simulink model "mCounterWithSaturation"  (R2021b)
settings: Solver=FixedStepAuto  StartTime=0.0  StopTime=10.0  RelTol=1e-3
PreLoadFcn:
  | A=1;B=1;C=2;D=1;
CloseFcn:
  | clear A B C D;
settings Model: Creator=nrangava  LastModifiedBy=nrangava
settings SolverCC: AlgebraicLoopSolver=TrustRegion  MaxZcPerStep=1
settings DataIOCC: SaveFormat=StructureWithTime  SaveState=on  DSMLogging=off  OutputSaveName=yout1,yout2
settings OptimizationCC: DefaultParameterBehavior=Inlined  EnhancedBackFolding=on  PassReuseOutputArgsAs=Individual arguments  ZeroExternalMemoryAtStartup=off  ZeroInternalMemoryAtStartup=off  OptimizeBlockOrder=speed  DifferentSizesBufferReuse=on  OptimizationCustomize=off  EfficientTunableParamExpr=on
settings DebuggingCC: ParameterTunabilityLossMsg=error  SFMachineParentedDataDiag=warning
settings HardwareCC: TargetBitPerPointer=64  TargetBitPerSizeT=64  TargetBitPerPtrDiffT=64  TargetLongLongMode=on  TargetIntDivRoundTo=Zero  TargetEndianess=LittleEndian  TargetWordSize=64  TargetHWDeviceType=Custom Processor->MATLAB Host Computer  ProdEqTarget=off
settings ModelReferenceCC: UpdateModelReferenceTargets=IfOutOfDate
settings SFSimCC: MATLABDynamicMemAlloc=off
settings RTWCC: Description=Embedded Coder  SystemTargetFile=ert.tlc  TemplateMakefile=ert_default_tmf  RTWVerbose=off  RetainRTWFile=on  TLCAssert=on
settings CodeAppCC: ForceParamTrailComments=on  IgnoreCustomStorageClasses=off  MaxIdLength=64  OperatorAnnotations=on  SimulinkDataObjDesc=on  SFDataObjDesc=on  InsertBlockDesc=on
settings ERTTargetCC: TargetLangStandard=C99 (ISO)  GenerateSampleERTMain=on  CombineOutputUpdateFcns=off  LogVarNameModifier=none  MatFileLogging=on  InlinedParameterPlacement=NonHierarchical  ERTCustomFileTemplate=example_file_process.tlc

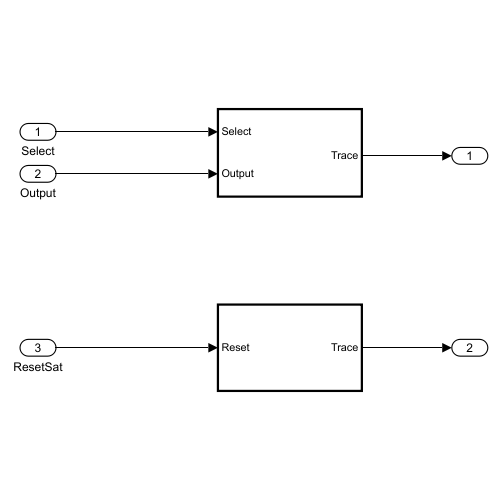
[thumbnail: Simulink's stored preview of the top-level diagram]
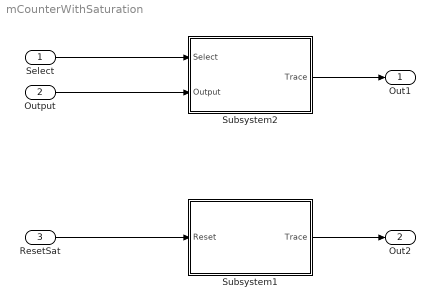
== system mCounterWithSaturation ==
  Select : Inport
  Output : Inport  Port=2
  ResetSat : Inport  Port=3  OutDataTypeStr=boolean
  Subsystem1 : Subsystem  TreatAsAtomicUnit=on  VariantControl=C==2
  Subsystem2 : Subsystem  TreatAsAtomicUnit=on  VariantControl=C==2
  Out1 : Outport
  Out2 : Outport  Port=2
  wires:
  ResetSat/1 -> Subsystem1/1(Reset)
  Select/1 -> Subsystem2/1(Select)
  Output/1 -> Subsystem2/2(Output)
  Subsystem2/1(Trace) -> Out1/1
  Subsystem1/1(Trace) -> Out2/1

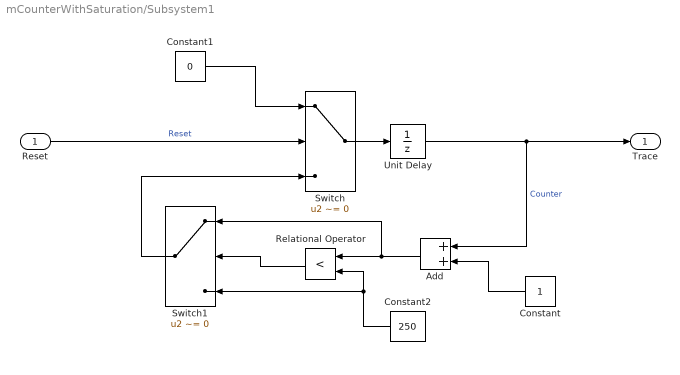
== system mCounterWithSaturation/Subsystem1 ==
  Reset : Inport
  Add : Sum
  Constant : Constant
  Constant1 : Constant  Value=0
  Constant2 : Constant  Value=250
  Relational Operator : RelationalOperator  Operator=<  OutDataTypeStr=boolean  RndMeth=Simplest
  Switch : Switch  Criteria=u2 ~= 0
  Switch1 : Switch  Criteria=u2 ~= 0
  Unit Delay : UnitDelay  SampleTime=-1  HasFrameUpgradeWarning=on
  Trace : Outport
  wires:
  Switch/1 -> Unit Delay/1
  Constant1/1 -> Switch/1
  Unit Delay/1 -> Trace/1, Add/1  "Counter"
  Constant/1 -> Add/2
  Reset/1 -> Switch/2  "Reset"
  Add/1 -> Switch1/1, Relational Operator/1
  Constant2/1 -> Switch1/3, Relational Operator/2
  Relational Operator/1 -> Switch1/2
  Switch1/1 -> Switch/3

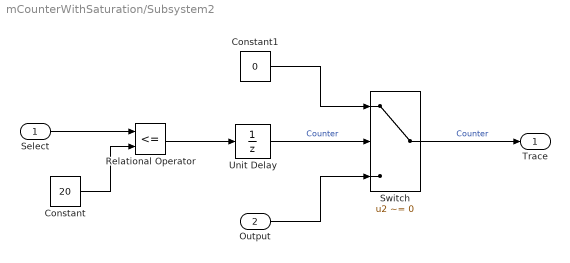
== system mCounterWithSaturation/Subsystem2 ==
  Select : Inport
  Output : Inport  Port=2
  Constant : Constant  Value=20
  Constant1 : Constant  Value=0
  Relational Operator : RelationalOperator  Operator=<=  OutDataTypeStr=boolean  RndMeth=Simplest
  Switch : Switch  Criteria=u2 ~= 0
  Unit Delay : UnitDelay  SampleTime=-1  HasFrameUpgradeWarning=on
  Trace : Outport
  wires:
  Switch/1 -> Trace/1  "Counter"
  Constant1/1 -> Switch/1
  Unit Delay/1 -> Switch/2  "Counter"
  Relational Operator/1 -> Unit Delay/1
  Select/1 -> Relational Operator/1
  Constant/1 -> Relational Operator/2
  Output/1 -> Switch/3
